simulink model "Crosquis_Salida_Conversor_simple_AC_DC"  (R2019b)
settings: Solver=VariableStepAuto  StartTime=0.0  StopTime=0.2  MaxStep=100e-6  RelTol=1e-3
settings Model: Creator=roger  LastModifiedBy=belindabrown
settings SFSimCC: CustomCodeUndefinedFunction=UseInterfaceOnly

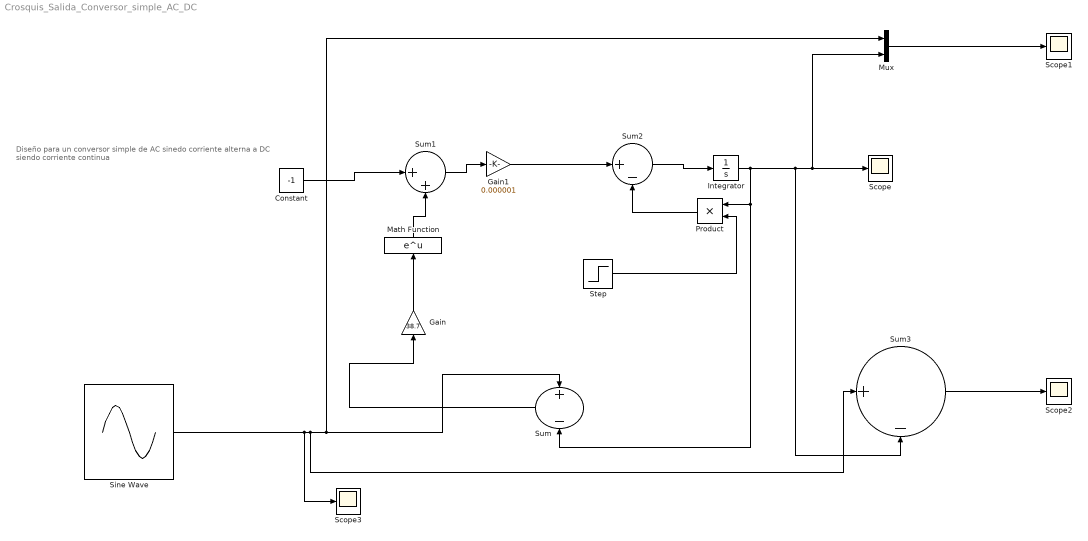
== system Crosquis_Salida_Conversor_simple_AC_DC ==
  note: Diseño para un conversor simple de AC sinedo corriente alterna a DC siendo corriente continua
  Constant : Constant  Value=-1
  Gain : Gain  Gain=38.7
  Gain1 : Gain  Gain=0.000001
  Integrator : Integrator
  Math Function : Math  SaturateOnIntegerOverflow=on
  Mux : Mux  Inputs=2
  Product : Product
  Scope{,1..3} (4 alike) : Scope
  Sine Wave : Sin  Amplitude=12  Frequency=2*pi*60  SampleTime=0
  Step : Step  Time=0.1  Before=10  After=40  SampleTime=0
  Sum : Sum  Inputs=+-
  Sum1 : Sum  Inputs=|++
  Sum2 : Sum  Inputs=|+-
  Sum3 : Sum  Inputs=|+-
  wires:
  Sine Wave/1 -> Scope3/1, Sum/1, Mux/1, Sum3/1
  Sum/1 -> Gain/1
  Gain/1 -> Math Function/1
  Math Function/1 -> Sum1/2
  Constant/1 -> Sum1/1
  Sum2/1 -> Integrator/1
  Integrator/1 -> Sum3/2, Mux/2, Scope/1, Product/1, Sum/2
  Mux/1 -> Scope1/1
  Sum3/1 -> Scope2/1
  Sum1/1 -> Gain1/1
  Gain1/1 -> Sum2/1
  Product/1 -> Sum2/2
  Step/1 -> Product/2
